simulink model "TestStructure"  (R2022b)
settings: Solver=FixedStepDiscrete  StartTime=0.0  StopTime=300  FixedStep=SampleTime  RelTol=1e-3
InitFcn:
  | SampleTime = 0.001;
  | ButtonValue=0;
  | load("BusConfig.mat");
model workspace (MAT data in the model file):
  Manual_Auto = 1
  Pattern = 1
  Pause_Start = 1
  Stop = 1
  Unlock_Lock = 1
undefined symbols (not defined in the file or in its folder): DiscIntNeverNeededParam
libraries: dspfdesign x4, dspstat3 x4
(part 2 of 3)

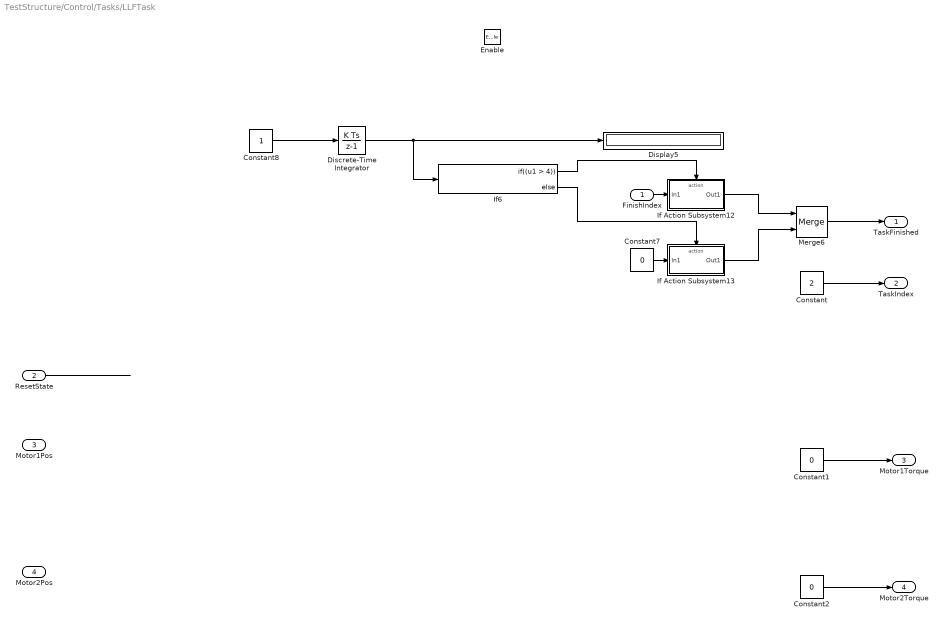
== system TestStructure/Control/Tasks/LLFTask ==
  FinishIndex : Inport
  ResetState : Inport  Port=2
  Motor1Pos : Inport  Port=3
  Motor2Pos : Inport  Port=4
  Enable : EnablePort  StatesWhenEnabling=reset
  Constant : Constant  Value=2
  Constant1 : Constant  Value=0
  Constant2 : Constant  Value=0
  Constant7 : Constant  Value=0  OutDataTypeStr=double
  Constant8 : Constant
  Discrete-Time Integrator : DiscreteIntegrator  SampleTime=-1  ICPrevOutput=DiscIntNeverNeededParam  ICPrevScaledInput=DiscIntNeverNeededParam
  Display5 : Display
  If Action Subsystem12 : Subsystem  TreatAsAtomicUnit=on
  If Action Subsystem13 : Subsystem  TreatAsAtomicUnit=on
  If6 : If  IfExpression=(u1 > 4)
  Merge6 : Merge
  TaskFinished : Outport
  TaskIndex : Outport  Port=2
  Motor1Torque : Outport  Port=3
  Motor2Torque : Outport  Port=4
  wires:
  Merge6/1 -> TaskFinished/1
  If6/1 -> If Action Subsystem12/Action
  Constant8/1 -> Discrete-Time Integrator/1
  If6/2 -> If Action Subsystem13/Action
  Discrete-Time Integrator/1 -> If6/1, Display5/1
  If Action Subsystem13/1(Out1) -> Merge6/2
  FinishIndex/1 -> If Action Subsystem12/1(In1)
  If Action Subsystem12/1(Out1) -> Merge6/1
  Constant7/1 -> If Action Subsystem13/1(In1)
  Constant/1 -> TaskIndex/1
  Constant1/1 -> Motor1Torque/1
  Constant2/1 -> Motor2Torque/1
  ResetState/1 -> ?

== system TestStructure/Control/Tasks/LLWAutoTask ==
  FinishIndex : Inport
  ResetState : Inport  Port=2
  Motor1Pos : Inport  Port=3
  Motor2Pos : Inport  Port=4
  Enable : EnablePort  StatesWhenEnabling=reset
  Constant : Constant  Value=8
  Constant1 : Constant  Value=0
  Constant2 : Constant  Value=0
  Constant7 : Constant  Value=0  OutDataTypeStr=double
  Constant8 : Constant
  Discrete-Time Integrator : DiscreteIntegrator  SampleTime=-1  ICPrevOutput=DiscIntNeverNeededParam  ICPrevScaledInput=DiscIntNeverNeededParam
  Display5 : Display
  If Action Subsystem12 : Subsystem  TreatAsAtomicUnit=on
  If Action Subsystem13 : Subsystem  TreatAsAtomicUnit=on
  If6 : If  IfExpression=(u1 > 4)
  Merge6 : Merge
  TaskFinished : Outport
  TaskIndex : Outport  Port=2
  Motor1Torque : Outport  Port=3
  Motor2Torque : Outport  Port=4
  wires:
  Merge6/1 -> TaskFinished/1
  If6/1 -> If Action Subsystem12/Action
  Constant8/1 -> Discrete-Time Integrator/1
  If6/2 -> If Action Subsystem13/Action
  Discrete-Time Integrator/1 -> If6/1, Display5/1
  If Action Subsystem13/1(Out1) -> Merge6/2
  FinishIndex/1 -> If Action Subsystem12/1(In1)
  If Action Subsystem12/1(Out1) -> Merge6/1
  Constant7/1 -> If Action Subsystem13/1(In1)
  Constant/1 -> TaskIndex/1
  Constant1/1 -> Motor1Torque/1
  Constant2/1 -> Motor2Torque/1
  ResetState/1 -> ?

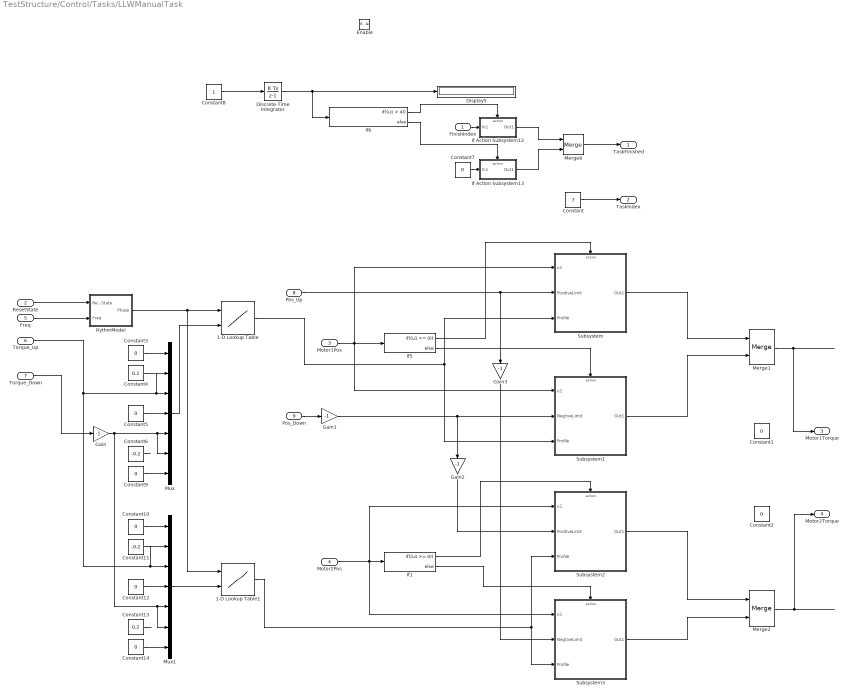
== system TestStructure/Control/Tasks/LLWManualTask ==
  FinishIndex : Inport
  ResetState : Inport  Port=2
  Motor1Pos : Inport  Port=3
  Motor2Pos : Inport  Port=4
  Freq : Inport  Port=5
  Torque_Up : Inport  Port=6
  Torque_Down : Inport  Port=7
  Pos_Up : Inport  Port=8
  Pos_Down : Inport  Port=9
  Enable : EnablePort
  1-D Lookup Table : Lookup_n-D  NumberOfTableDimensions=1  BreakpointsForDimension1=[0;0.2;0.35;0.5;0.65;0.85;1]  TableSource=Input port  Table=[0;0.2;3;0;-3;-0.2;0]  InternalRulePriority=Speed  RndMeth=Simplest
      settings: InputPortMap=u0,p221
  1-D Lookup Table1 : Lookup_n-D  NumberOfTableDimensions=1  BreakpointsForDimension1=[0;0.2;0.35;0.5;0.65;0.85;1]  TableSource=Input port  Table=[0;0.2;3;0;-3;-0.2;0]  InternalRulePriority=Speed  RndMeth=Simplest
      settings: InputPortMap=u0,p221
  Constant : Constant  Value=7
  Constant{1..3,5,9..10,12,14} (8 alike) : Constant  Value=0
  Constant11 : Constant  Value=-0.2
  Constant13 : Constant  Value=0.2
  Constant4 : Constant  Value=0.2
  Constant6 : Constant  Value=-0.2
  Constant7 : Constant  Value=0  OutDataTypeStr=double
  Constant8 : Constant
  Discrete-Time Integrator : DiscreteIntegrator  SampleTime=-1  ICPrevOutput=DiscIntNeverNeededParam  ICPrevScaledInput=DiscIntNeverNeededParam
  Display5 : Display
  Gain{,1..3} (4 alike) : Gain  Gain=-1
  If Action Subsystem12 : Subsystem  TreatAsAtomicUnit=on
  If Action Subsystem13 : Subsystem  TreatAsAtomicUnit=on
  If1 : If  IfExpression=(u1 >= 0)
  If5 : If  IfExpression=(u1 >= 0)
  If6 : If  IfExpression=(u1 > 4)
  Merge1 : Merge
  Merge2 : Merge
  Merge6 : Merge
  Mux : Mux  Inputs=7
  Mux1 : Mux  Inputs=7
  RythmModel : Subsystem
  Subsystem : Subsystem
  Subsystem1 : Subsystem
  Subsystem2 : Subsystem
  Subsystem3 : Subsystem
  TaskFinished : Outport
  TaskIndex : Outport  Port=2
  Motor1Torque : Outport  Port=3
  Motor2Torque : Outport  Port=4
  wires:
  Merge6/1 -> TaskFinished/1
  If6/1 -> If Action Subsystem12/Action
  Constant8/1 -> Discrete-Time Integrator/1
  If6/2 -> If Action Subsystem13/Action
  Discrete-Time Integrator/1 -> If6/1, Display5/1
  If Action Subsystem13/1(Out1) -> Merge6/2
  FinishIndex/1 -> If Action Subsystem12/1(In1)
  If Action Subsystem12/1(Out1) -> Merge6/1
  Constant7/1 -> If Action Subsystem13/1(In1)
  Constant/1 -> TaskIndex/1
  If5/1 -> Subsystem/Action
  Mux1/1 -> 1-D Lookup Table1/2
  Gain3/1 -> Subsystem3/2(NegtiveLimit)
  1-D Lookup Table1/1 -> Subsystem2/3(Profile), Subsystem3/3(Profile)
  Constant12/1 -> Mux1/4
  1-D Lookup Table/1 -> Subsystem1/3(Profile), Subsystem/3(Profile)
  Subsystem/1(Out1) -> Merge1/1
  Mux/1 -> 1-D Lookup Table/2
  Merge1/1 -> Motor1Torque/1
  Merge2/1 -> Motor2Torque/1
  If5/2 -> Subsystem1/Action
  Gain2/1 -> Subsystem2/2(PositiveLimit)
  Gain/1 -> Mux1/5, Mux1/6, Mux/6, Mux/5
  Constant3/1 -> Mux/1
  If1/2 -> Subsystem3/Action
  Subsystem2/1(Out1) -> Merge2/1
  Constant10/1 -> Mux1/1
  Constant5/1 -> Mux/4
  Constant14/1 -> Mux1/7
  ResetState/1 -> RythmModel/1(ResetState)
  Pos_Down/1 -> Gain1/1
  Subsystem1/1(Out1) -> Merge1/2
  If1/1 -> Subsystem2/Action
  RythmModel/1(Phase) -> 1-D Lookup Table1/1, 1-D Lookup Table/1
  Torque_Up/1 -> Mux1/2, Mux1/3, Mux/2, Mux/3
  Subsystem3/1(Out1) -> Merge2/2
  Constant9/1 -> Mux/7
  Constant6/1 -> ?
  Motor1Pos/1 -> Subsystem1/1(u1), If5/1, Subsystem/1(u1)
  Constant13/1 -> ?
  Freq/1 -> RythmModel/2(Freq)
  Torque_Down/1 -> Gain/1
  Constant11/1 -> ?
  Motor2Pos/1 -> Subsystem3/1(u1), Subsystem2/1(u1), If1/1
  Gain1/1 -> Subsystem1/2(NegtiveLimit), Gain2/1
  Constant4/1 -> ?
  Pos_Up/1 -> Subsystem/2(PositiveLimit), Gain3/1

== system TestStructure/Control/Tasks/PauseTask ==
  FinishIndex : Inport
  ResetState : Inport  Port=2
  Motor1Pos : Inport  Port=3
  Motor2Pos : Inport  Port=4
  Enable : EnablePort  StatesWhenEnabling=reset
  Constant : Constant  Value=9
  Constant1 : Constant  Value=0
  Constant2 : Constant  Value=0
  Constant7 : Constant  Value=0  OutDataTypeStr=double
  Constant8 : Constant
  Discrete-Time Integrator : DiscreteIntegrator  SampleTime=-1  ICPrevOutput=DiscIntNeverNeededParam  ICPrevScaledInput=DiscIntNeverNeededParam
  Display5 : Display
  If Action Subsystem12 : Subsystem  TreatAsAtomicUnit=on
  If Action Subsystem13 : Subsystem  TreatAsAtomicUnit=on
  If6 : If  IfExpression=(u1 > 4)
  Merge6 : Merge
  TaskFinished : Outport
  TaskIndex : Outport  Port=2
  Motor1Torque : Outport  Port=3
  Motor2Torque : Outport  Port=4
  wires:
  Merge6/1 -> TaskFinished/1
  If6/1 -> If Action Subsystem12/Action
  Constant8/1 -> Discrete-Time Integrator/1
  If6/2 -> If Action Subsystem13/Action
  Discrete-Time Integrator/1 -> If6/1, Display5/1
  If Action Subsystem13/1(Out1) -> Merge6/2
  FinishIndex/1 -> If Action Subsystem12/1(In1)
  If Action Subsystem12/1(Out1) -> Merge6/1
  Constant7/1 -> If Action Subsystem13/1(In1)
  Constant/1 -> TaskIndex/1
  Constant1/1 -> Motor1Torque/1
  Constant2/1 -> Motor2Torque/1
  ResetState/1 -> ?

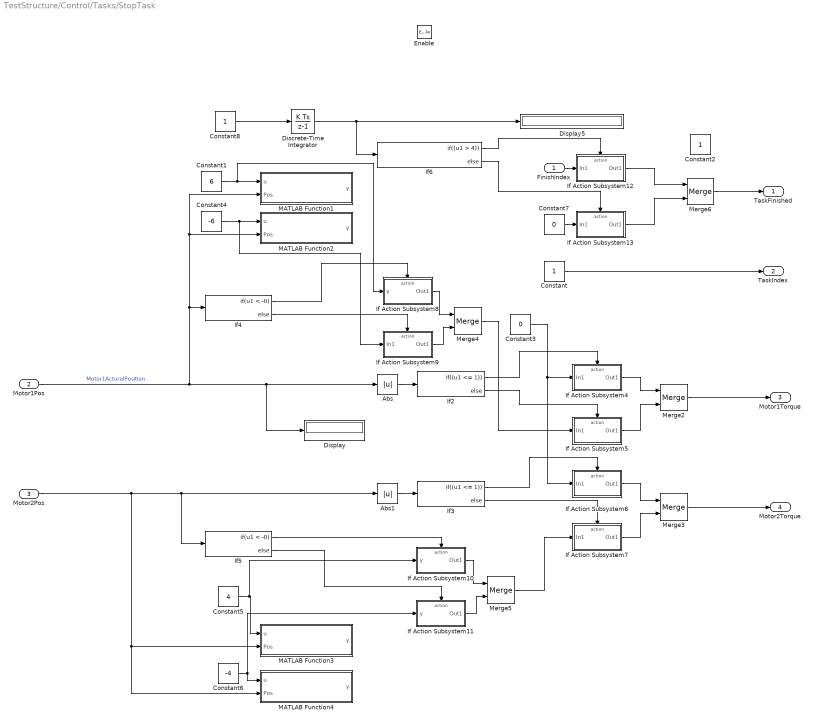
== system TestStructure/Control/Tasks/StopTask ==
  FinishIndex : Inport
  Motor1Pos : Inport  Port=2
  Motor2Pos : Inport  Port=3
  Enable : EnablePort  StatesWhenEnabling=reset
  Abs : Abs  SaturateOnIntegerOverflow=off
  Abs1 : Abs  SaturateOnIntegerOverflow=off
  Constant : Constant
  Constant1 : Constant  Value=6
  Constant2 : Constant
  Constant3 : Constant  Value=0
  Constant4 : Constant  Value=-6
  Constant5 : Constant  Value=4
  Constant6 : Constant  Value=-4
  Constant7 : Constant  Value=0  OutDataTypeStr=double
  Constant8 : Constant
  Discrete-Time Integrator : DiscreteIntegrator  SampleTime=-1  ICPrevOutput=DiscIntNeverNeededParam  ICPrevScaledInput=DiscIntNeverNeededParam
  Display : Display
  Display5 : Display
  If Action Subsystem10 : Subsystem  TreatAsAtomicUnit=on
  If Action Subsystem11 : Subsystem  TreatAsAtomicUnit=on
  If Action Subsystem12 : Subsystem  TreatAsAtomicUnit=on
  If Action Subsystem13 : Subsystem  TreatAsAtomicUnit=on
  If Action Subsystem4 : Subsystem  TreatAsAtomicUnit=on
  If Action Subsystem5 : Subsystem  TreatAsAtomicUnit=on
  If Action Subsystem6 : Subsystem  TreatAsAtomicUnit=on
  If Action Subsystem7 : Subsystem  TreatAsAtomicUnit=on
  If Action Subsystem8 : Subsystem  TreatAsAtomicUnit=on
  If Action Subsystem9 : Subsystem  TreatAsAtomicUnit=on
  If2 : If  IfExpression=(u1 <= 1)
  If3 : If  IfExpression=(u1 <= 1)
  If4 : If  IfExpression=u1 < -0
  If5 : If  IfExpression=u1 < -0
  If6 : If  IfExpression=(u1 > 4)
  MATLAB Function1 : MATLAB Function  TreatAsAtomicUnit=on
  MATLAB Function2 : MATLAB Function  TreatAsAtomicUnit=on
  MATLAB Function3 : MATLAB Function  TreatAsAtomicUnit=on
  MATLAB Function4 : MATLAB Function  TreatAsAtomicUnit=on
  Merge{2..6} (5 alike) : Merge
  TaskFinished : Outport
  TaskIndex : Outport  Port=2
  Motor1Torque : Outport  Port=3
  Motor2Torque : Outport  Port=4
  wires:
  Merge6/1 -> TaskFinished/1
  If6/1 -> If Action Subsystem12/Action
  If2/1 -> If Action Subsystem4/Action
  Constant1/1 -> If Action Subsystem8/1(y), MATLAB Function1/1(u)
  If Action Subsystem11/1(Out1) -> Merge5/2
  Constant5/1 -> If Action Subsystem10/1(y), MATLAB Function3/1(u)
  If5/2 -> If Action Subsystem11/Action
  If4/2 -> If Action Subsystem9/Action
  If Action Subsystem8/1(Out1) -> Merge4/1
  If3/2 -> If Action Subsystem7/Action
  If4/1 -> If Action Subsystem8/Action
  If Action Subsystem10/1(Out1) -> Merge5/1
  Constant8/1 -> Discrete-Time Integrator/1
  If2/2 -> If Action Subsystem5/Action
  Merge5/1 -> If Action Subsystem7/1(In1)
  Merge3/1 -> Motor2Torque/1
  If5/1 -> If Action Subsystem10/Action
  Abs/1 -> If2/1
  Merge4/1 -> If Action Subsystem5/1(In1)
  Merge2/1 -> Motor1Torque/1
  Constant3/1 -> If Action Subsystem6/1(In1), If Action Subsystem4/1(In1)
  If Action Subsystem9/1(Out1) -> Merge4/2
  Motor2Pos/1 -> MATLAB Function4/2(Pos), MATLAB Function3/2(Pos), If5/1, Abs1/1
  Motor1Pos/1 -> MATLAB Function2/2(Pos), MATLAB Function1/2(Pos), If4/1, Abs/1, Display/1  "Motor1ActuralPosition"
  If6/2 -> If Action Subsystem13/Action
  Abs1/1 -> If3/1
  Discrete-Time Integrator/1 -> If6/1, Display5/1
  If Action Subsystem13/1(Out1) -> Merge6/2
  If Action Subsystem7/1(Out1) -> Merge3/2
  FinishIndex/1 -> If Action Subsystem12/1(In1)
  If Action Subsystem12/1(Out1) -> Merge6/1
  If Action Subsystem6/1(Out1) -> Merge3/1
  If Action Subsystem4/1(Out1) -> Merge2/1
  If3/1 -> If Action Subsystem6/Action
  If Action Subsystem5/1(Out1) -> Merge2/2
  Constant7/1 -> If Action Subsystem13/1(In1)
  Constant4/1 -> If Action Subsystem9/1(In1), MATLAB Function2/1(u)
  Constant6/1 -> If Action Subsystem11/1(y), MATLAB Function4/1(u)
  Constant/1 -> TaskIndex/1

== system TestStructure/Control/Tasks/ULLockTask ==
  FinishIndex : Inport
  ResetState : Inport  Port=2
  Motor3Pos : Inport  Port=3
  Motor4Pos : Inport  Port=4
  Enable : EnablePort  StatesWhenEnabling=reset
  Constant : Constant  Value=2
  Constant1 : Constant  Value=0
  Constant2 : Constant  Value=0
  Constant7 : Constant  Value=0  OutDataTypeStr=double
  Constant8 : Constant
  Discrete-Time Integrator : DiscreteIntegrator  SampleTime=-1  ICPrevOutput=DiscIntNeverNeededParam  ICPrevScaledInput=DiscIntNeverNeededParam
  Display5 : Display
  If Action Subsystem12 : Subsystem  TreatAsAtomicUnit=on
  If Action Subsystem13 : Subsystem  TreatAsAtomicUnit=on
  If6 : If  IfExpression=(u1 > 4)
  Merge6 : Merge
  TaskFinished : Outport
  TaskIndex : Outport  Port=2
  Motor3Torque : Outport  Port=3
  Motor4Torque : Outport  Port=4
  wires:
  Merge6/1 -> TaskFinished/1
  If6/1 -> If Action Subsystem12/Action
  Constant8/1 -> Discrete-Time Integrator/1
  If6/2 -> If Action Subsystem13/Action
  Discrete-Time Integrator/1 -> If6/1, Display5/1
  If Action Subsystem13/1(Out1) -> Merge6/2
  FinishIndex/1 -> If Action Subsystem12/1(In1)
  If Action Subsystem12/1(Out1) -> Merge6/1
  Constant7/1 -> If Action Subsystem13/1(In1)
  Constant/1 -> TaskIndex/1
  Constant1/1 -> Motor3Torque/1
  Constant2/1 -> Motor4Torque/1
  ResetState/1 -> ?

== system TestStructure/Control/Tasks/ULUnLockTask ==
  FinishIndex : Inport
  ResetState : Inport  Port=2
  Motor3Pos : Inport  Port=3
  Motor4Pos : Inport  Port=4
  Enable : EnablePort  StatesWhenEnabling=reset
  Constant : Constant
  Constant1 : Constant  Value=0
  Constant2 : Constant  Value=0
  Constant7 : Constant  Value=0  OutDataTypeStr=double
  Constant8 : Constant
  Discrete-Time Integrator : DiscreteIntegrator  SampleTime=-1  ICPrevOutput=DiscIntNeverNeededParam  ICPrevScaledInput=DiscIntNeverNeededParam
  Display5 : Display
  If Action Subsystem12 : Subsystem  TreatAsAtomicUnit=on
  If Action Subsystem13 : Subsystem  TreatAsAtomicUnit=on
  If6 : If  IfExpression=(u1 > 4)
  Merge6 : Merge
  TaskFinished : Outport
  TaskIndex : Outport  Port=2
  Motor3Torque : Outport  Port=3
  Motor4Torque : Outport  Port=4
  wires:
  Merge6/1 -> TaskFinished/1
  If6/1 -> If Action Subsystem12/Action
  Constant8/1 -> Discrete-Time Integrator/1
  If6/2 -> If Action Subsystem13/Action
  Discrete-Time Integrator/1 -> If6/1, Display5/1
  If Action Subsystem13/1(Out1) -> Merge6/2
  FinishIndex/1 -> If Action Subsystem12/1(In1)
  If Action Subsystem12/1(Out1) -> Merge6/1
  Constant7/1 -> If Action Subsystem13/1(In1)
  Constant/1 -> TaskIndex/1
  Constant1/1 -> Motor3Torque/1
  Constant2/1 -> Motor4Torque/1
  ResetState/1 -> ?

== system TestStructure/Control/PanelController/Display_State_1_Enable/Subsystem ==
  Case : Inport
  Case Default : Inport  Port=2
  Constant : Constant
  Constant1 : Constant  Value=0
  Constant2 : Constant  Value=TaskIndex
  Merge : Merge
  Switch Case Action Subsystem : Subsystem  TreatAsAtomicUnit=on
  Switch Case Action Subsystem1 : Subsystem  TreatAsAtomicUnit=on
  Enable : Outport
  FinishIndex : Outport  Port=2
  wires:
  Constant/1 -> Switch Case Action Subsystem/1(In1)
  Case/1 -> Switch Case Action Subsystem/Action
  Switch Case Action Subsystem/1(Out1) -> Merge/1
  Merge/1 -> Enable/1
  Case Default/1 -> Switch Case Action Subsystem1/Action
  Constant1/1 -> Switch Case Action Subsystem1/1(In1)
  Switch Case Action Subsystem1/1(Default) -> Merge/2
  Constant2/1 -> FinishIndex/1

== system TestStructure/Control/PanelController/Display_State_2_Enable/Subsystem ==
  Case : Inport
  Case Default : Inport  Port=2
  Constant : Constant
  Constant1 : Constant  Value=0
  Constant2 : Constant  Value=TaskIndex
  Merge : Merge
  Switch Case Action Subsystem : Subsystem  TreatAsAtomicUnit=on
  Switch Case Action Subsystem1 : Subsystem  TreatAsAtomicUnit=on
  Enable : Outport
  FinishIndex : Outport  Port=2
  wires:
  Constant/1 -> Switch Case Action Subsystem/1(In1)
  Case/1 -> Switch Case Action Subsystem/Action
  Switch Case Action Subsystem/1(Out1) -> Merge/1
  Merge/1 -> Enable/1
  Case Default/1 -> Switch Case Action Subsystem1/Action
  Constant1/1 -> Switch Case Action Subsystem1/1(In1)
  Switch Case Action Subsystem1/1(Default) -> Merge/2
  Constant2/1 -> FinishIndex/1

== system TestStructure/Control/PanelController/Display_State_3_Enable/Subsystem ==
  Case : Inport
  Case Default : Inport  Port=2
  Constant : Constant
  Constant1 : Constant  Value=0
  Constant2 : Constant  Value=TaskIndex
  Merge : Merge
  Switch Case Action Subsystem : Subsystem  TreatAsAtomicUnit=on
  Switch Case Action Subsystem1 : Subsystem  TreatAsAtomicUnit=on
  Enable : Outport
  FinishIndex : Outport  Port=2
  wires:
  Constant/1 -> Switch Case Action Subsystem/1(In1)
  Case/1 -> Switch Case Action Subsystem/Action
  Switch Case Action Subsystem/1(Out1) -> Merge/1
  Merge/1 -> Enable/1
  Case Default/1 -> Switch Case Action Subsystem1/Action
  Constant1/1 -> Switch Case Action Subsystem1/1(In1)
  Switch Case Action Subsystem1/1(Default) -> Merge/2
  Constant2/1 -> FinishIndex/1

== system TestStructure/Control/PanelController/Display_State_4_Enable/Subsystem ==
  Case : Inport
  Case Default : Inport  Port=2
  Constant : Constant
  Constant1 : Constant  Value=0
  Constant2 : Constant  Value=TaskIndex
  Merge : Merge
  Switch Case Action Subsystem : Subsystem  TreatAsAtomicUnit=on
  Switch Case Action Subsystem1 : Subsystem  TreatAsAtomicUnit=on
  Enable : Outport
  FinishIndex : Outport  Port=2
  wires:
  Constant/1 -> Switch Case Action Subsystem/1(In1)
  Case/1 -> Switch Case Action Subsystem/Action
  Switch Case Action Subsystem/1(Out1) -> Merge/1
  Merge/1 -> Enable/1
  Case Default/1 -> Switch Case Action Subsystem1/Action
  Constant1/1 -> Switch Case Action Subsystem1/1(In1)
  Switch Case Action Subsystem1/1(Default) -> Merge/2
  Constant2/1 -> FinishIndex/1

== system TestStructure/Control/PanelController/LLTaskControl_State_1_Enable/Subsystem ==
  Case : Inport
  Case Default : Inport  Port=2
  Constant : Constant
  Constant1 : Constant  Value=0
  Constant2 : Constant  Value=TaskIndex
  Merge : Merge
  Switch Case Action Subsystem : Subsystem  TreatAsAtomicUnit=on
  Switch Case Action Subsystem1 : Subsystem  TreatAsAtomicUnit=on
  Enable : Outport
  FinishIndex : Outport  Port=2
  wires:
  Constant/1 -> Switch Case Action Subsystem/1(In1)
  Case/1 -> Switch Case Action Subsystem/Action
  Switch Case Action Subsystem/1(Out1) -> Merge/1
  Merge/1 -> Enable/1
  Case Default/1 -> Switch Case Action Subsystem1/Action
  Constant1/1 -> Switch Case Action Subsystem1/1(In1)
  Switch Case Action Subsystem1/1(Default) -> Merge/2
  Constant2/1 -> FinishIndex/1

== system TestStructure/Control/PanelController/LLTaskControl_State_2_Enable/Subsystem ==
  Case : Inport
  Case Default : Inport  Port=2
  Constant : Constant
  Constant1 : Constant  Value=0
  Constant2 : Constant  Value=TaskIndex
  Merge : Merge
  Switch Case Action Subsystem : Subsystem  TreatAsAtomicUnit=on
  Switch Case Action Subsystem1 : Subsystem  TreatAsAtomicUnit=on
  Enable : Outport
  FinishIndex : Outport  Port=2
  wires:
  Constant/1 -> Switch Case Action Subsystem/1(In1)
  Case/1 -> Switch Case Action Subsystem/Action
  Switch Case Action Subsystem/1(Out1) -> Merge/1
  Merge/1 -> Enable/1
  Case Default/1 -> Switch Case Action Subsystem1/Action
  Constant1/1 -> Switch Case Action Subsystem1/1(In1)
  Switch Case Action Subsystem1/1(Default) -> Merge/2
  Constant2/1 -> FinishIndex/1

== system TestStructure/Control/PanelController/LLTaskControl_State_3_Enable/Subsystem ==
  Case : Inport
  Case Default : Inport  Port=2
  Constant : Constant
  Constant1 : Constant  Value=0
  Constant2 : Constant  Value=TaskIndex
  Merge : Merge
  Switch Case Action Subsystem : Subsystem  TreatAsAtomicUnit=on
  Switch Case Action Subsystem1 : Subsystem  TreatAsAtomicUnit=on
  Enable : Outport
  FinishIndex : Outport  Port=2
  wires:
  Constant/1 -> Switch Case Action Subsystem/1(In1)
  Case/1 -> Switch Case Action Subsystem/Action
  Switch Case Action Subsystem/1(Out1) -> Merge/1
  Merge/1 -> Enable/1
  Case Default/1 -> Switch Case Action Subsystem1/Action
  Constant1/1 -> Switch Case Action Subsystem1/1(In1)
  Switch Case Action Subsystem1/1(Default) -> Merge/2
  Constant2/1 -> FinishIndex/1

== system TestStructure/Control/PanelController/LLTaskControl_State_4_Enable/Subsystem ==
  Case : Inport
  Case Default : Inport  Port=2
  Constant : Constant
  Constant1 : Constant  Value=0
  Constant2 : Constant  Value=TaskIndex
  Merge : Merge
  Switch Case Action Subsystem : Subsystem  TreatAsAtomicUnit=on
  Switch Case Action Subsystem1 : Subsystem  TreatAsAtomicUnit=on
  Enable : Outport
  FinishIndex : Outport  Port=2
  wires:
  Constant/1 -> Switch Case Action Subsystem/1(In1)
  Case/1 -> Switch Case Action Subsystem/Action
  Switch Case Action Subsystem/1(Out1) -> Merge/1
  Merge/1 -> Enable/1
  Case Default/1 -> Switch Case Action Subsystem1/Action
  Constant1/1 -> Switch Case Action Subsystem1/1(In1)
  Switch Case Action Subsystem1/1(Default) -> Merge/2
  Constant2/1 -> FinishIndex/1

== system TestStructure/Control/PanelController/LLTaskControl_State_5_Enable/Subsystem ==
  Case : Inport
  Case Default : Inport  Port=2
  Constant : Constant
  Constant1 : Constant  Value=0
  Constant2 : Constant  Value=TaskIndex
  Merge : Merge
  Switch Case Action Subsystem : Subsystem  TreatAsAtomicUnit=on
  Switch Case Action Subsystem1 : Subsystem  TreatAsAtomicUnit=on
  Enable : Outport
  FinishIndex : Outport  Port=2
  wires:
  Constant/1 -> Switch Case Action Subsystem/1(In1)
  Case/1 -> Switch Case Action Subsystem/Action
  Switch Case Action Subsystem/1(Out1) -> Merge/1
  Merge/1 -> Enable/1
  Case Default/1 -> Switch Case Action Subsystem1/Action
  Constant1/1 -> Switch Case Action Subsystem1/1(In1)
  Switch Case Action Subsystem1/1(Default) -> Merge/2
  Constant2/1 -> FinishIndex/1

== system TestStructure/Control/PanelController/LLTaskControl_State_6_Enable/Subsystem ==
  Case : Inport
  Case Default : Inport  Port=2
  Constant : Constant
  Constant1 : Constant  Value=0
  Constant2 : Constant  Value=TaskIndex
  Merge : Merge
  Switch Case Action Subsystem : Subsystem  TreatAsAtomicUnit=on
  Switch Case Action Subsystem1 : Subsystem  TreatAsAtomicUnit=on
  Enable : Outport
  FinishIndex : Outport  Port=2
  wires:
  Constant/1 -> Switch Case Action Subsystem/1(In1)
  Case/1 -> Switch Case Action Subsystem/Action
  Switch Case Action Subsystem/1(Out1) -> Merge/1
  Merge/1 -> Enable/1
  Case Default/1 -> Switch Case Action Subsystem1/Action
  Constant1/1 -> Switch Case Action Subsystem1/1(In1)
  Switch Case Action Subsystem1/1(Default) -> Merge/2
  Constant2/1 -> FinishIndex/1

== system TestStructure/Control/PanelController/LLTaskControl_State_7_Enable/Subsystem ==
  Case : Inport
  Case Default : Inport  Port=2
  Constant : Constant
  Constant1 : Constant  Value=0
  Constant2 : Constant  Value=TaskIndex
  Merge : Merge
  Switch Case Action Subsystem : Subsystem  TreatAsAtomicUnit=on
  Switch Case Action Subsystem1 : Subsystem  TreatAsAtomicUnit=on
  Enable : Outport
  FinishIndex : Outport  Port=2
  wires:
  Constant/1 -> Switch Case Action Subsystem/1(In1)
  Case/1 -> Switch Case Action Subsystem/Action
  Switch Case Action Subsystem/1(Out1) -> Merge/1
  Merge/1 -> Enable/1
  Case Default/1 -> Switch Case Action Subsystem1/Action
  Constant1/1 -> Switch Case Action Subsystem1/1(In1)
  Switch Case Action Subsystem1/1(Default) -> Merge/2
  Constant2/1 -> FinishIndex/1

== system TestStructure/Control/PanelController/LLTaskControl_State_8_Enable/Subsystem ==
  Case : Inport
  Case Default : Inport  Port=2
  Constant : Constant
  Constant1 : Constant  Value=0
  Constant2 : Constant  Value=TaskIndex
  Merge : Merge
  Switch Case Action Subsystem : Subsystem  TreatAsAtomicUnit=on
  Switch Case Action Subsystem1 : Subsystem  TreatAsAtomicUnit=on
  Enable : Outport
  FinishIndex : Outport  Port=2
  wires:
  Constant/1 -> Switch Case Action Subsystem/1(In1)
  Case/1 -> Switch Case Action Subsystem/Action
  Switch Case Action Subsystem/1(Out1) -> Merge/1
  Merge/1 -> Enable/1
  Case Default/1 -> Switch Case Action Subsystem1/Action
  Constant1/1 -> Switch Case Action Subsystem1/1(In1)
  Switch Case Action Subsystem1/1(Default) -> Merge/2
  Constant2/1 -> FinishIndex/1

== system TestStructure/Control/PanelController/LLTaskControl_State_9_Enable/Subsystem ==
  Case : Inport
  Case Default : Inport  Port=2
  Constant : Constant
  Constant1 : Constant  Value=0
  Constant2 : Constant  Value=TaskIndex
  Merge : Merge
  Switch Case Action Subsystem : Subsystem  TreatAsAtomicUnit=on
  Switch Case Action Subsystem1 : Subsystem  TreatAsAtomicUnit=on
  Enable : Outport
  FinishIndex : Outport  Port=2
  wires:
  Constant/1 -> Switch Case Action Subsystem/1(In1)
  Case/1 -> Switch Case Action Subsystem/Action
  Switch Case Action Subsystem/1(Out1) -> Merge/1
  Merge/1 -> Enable/1
  Case Default/1 -> Switch Case Action Subsystem1/Action
  Constant1/1 -> Switch Case Action Subsystem1/1(In1)
  Switch Case Action Subsystem1/1(Default) -> Merge/2
  Constant2/1 -> FinishIndex/1

== system TestStructure/Control/PanelController/ULTaskControl_State_1_Enable/Subsystem ==
  Case : Inport
  Case Default : Inport  Port=2
  Constant : Constant
  Constant1 : Constant  Value=0
  Constant2 : Constant  Value=TaskIndex
  Merge : Merge
  Switch Case Action Subsystem : Subsystem  TreatAsAtomicUnit=on
  Switch Case Action Subsystem1 : Subsystem  TreatAsAtomicUnit=on
  Enable : Outport
  FinishIndex : Outport  Port=2
  wires:
  Constant/1 -> Switch Case Action Subsystem/1(In1)
  Case/1 -> Switch Case Action Subsystem/Action
  Switch Case Action Subsystem/1(Out1) -> Merge/1
  Merge/1 -> Enable/1
  Case Default/1 -> Switch Case Action Subsystem1/Action
  Constant1/1 -> Switch Case Action Subsystem1/1(In1)
  Switch Case Action Subsystem1/1(Default) -> Merge/2
  Constant2/1 -> FinishIndex/1

== system TestStructure/Control/PanelController/ULTaskControl_State_2_Enable/Subsystem ==
  Case : Inport
  Case Default : Inport  Port=2
  Constant : Constant
  Constant1 : Constant  Value=0
  Constant2 : Constant  Value=TaskIndex
  Merge : Merge
  Switch Case Action Subsystem : Subsystem  TreatAsAtomicUnit=on
  Switch Case Action Subsystem1 : Subsystem  TreatAsAtomicUnit=on
  Enable : Outport
  FinishIndex : Outport  Port=2
  wires:
  Constant/1 -> Switch Case Action Subsystem/1(In1)
  Case/1 -> Switch Case Action Subsystem/Action
  Switch Case Action Subsystem/1(Out1) -> Merge/1
  Merge/1 -> Enable/1
  Case Default/1 -> Switch Case Action Subsystem1/Action
  Constant1/1 -> Switch Case Action Subsystem1/1(In1)
  Switch Case Action Subsystem1/1(Default) -> Merge/2
  Constant2/1 -> FinishIndex/1

== system TestStructure/Control/Tasks/LLBAutoTask/If Action Subsystem12 ==
  In1 : Inport
  Action Port : ActionPort  ActionPortLabel=if((u1 > 4))
  Out1 : Outport
  wires:
  In1/1 -> Out1/1

== system TestStructure/Control/Tasks/LLBAutoTask/If Action Subsystem13 ==
  In1 : Inport
  Action Port : ActionPort  ActionPortLabel=else
  Out1 : Outport
  wires:
  In1/1 -> Out1/1

== system TestStructure/Control/Tasks/LLBManualTask/If Action Subsystem12 ==
  In1 : Inport
  Action Port : ActionPort  ActionPortLabel=if((u1 > 4))
  Out1 : Outport
  wires:
  In1/1 -> Out1/1

== system TestStructure/Control/Tasks/LLBManualTask/If Action Subsystem13 ==
  In1 : Inport
  Action Port : ActionPort  ActionPortLabel=else
  Out1 : Outport
  wires:
  In1/1 -> Out1/1

== system TestStructure/Control/Tasks/LLBManualTask/RythmModel ==
  ResetState : Inport
  Freq : Inport  Port=2
  Chart : Stateflow chart  TreatAsAtomicUnit=on
      settings: PortSchema="{\"entries\":[{\"content\":{\"sides\":[{\"content\":{\"connectorIds\":[\"In2\",\"In3\"]},\"type\":\"ConnectorPlacement.EquallySpacedRectSide\",\"uuid\":\"12385952-88cf-46bd-a9c8-6e14cd4b2c44\"},{\"content\":{\"connectorIds\":[\"Out1\",\"Out2\"],\"side\":\"RIGHT\"},\"type\":\"ConnectorPlacement.EquallySpacedRectSide\",\"uuid\":\"6211c7ba-d55b-4eba-bf5b-7c1649feb09f\"},{\"content\":{\"connectorIds\":[\"In1\"],\"side\":\"TOP\"},\"type\":\"ConnectorPlacement.EquallySpacedRectSide\",\"uuid\":\"17e15bab-f9dc-4c89-b15c-8ab250c59318\"},{\"content\":{\"connectorIds\":[\"In4\"],\"side\":\"BOTTOM\"},\"type\":\"ConnectorPlacement.EquallySpacedRectSide\",\"uuid\":\"029db472-06b3-40cc-b087-bfb8d6677823\"}]},\"type\":\"ConnectorPlacement.EquallySpacedConnector\",\"uuid\":\"9e8824a0-257a-42b2-87f9-63b657fce5f4\"}],\"packageUris\":[\"http://schema.mathworks.com/mf0/Connector/R2020b\"],\"version\":\"1.0\"}"
  Constant3 : Constant  Value=SampleTime
  Discrete-Time Integrator1 : DiscreteIntegrator  ExternalReset=rising  SampleTime=-1  LimitOutput=on  UpperSaturationLimit=1  LowerSaturationLimit=0  ICPrevOutput=DiscIntNeverNeededParam  ICPrevScaledInput=DiscIntNeverNeededParam
  Math Function : Math  Operator=reciprocal
  Memory : Memory
  Phase : Outport
  wires:
  Constant3/1 -> Chart/3(SampleTime)
  Discrete-Time Integrator1/1 -> Phase/1, Memory/1
  Chart/1(Input) -> Discrete-Time Integrator1/1
  Chart/2(Reset) -> Discrete-Time Integrator1/2
  Math Function/1 -> Chart/2(Period)
  Freq/1 -> Math Function/1
  Memory/1 -> Chart/4(IntVal)
  ResetState/1 -> Chart/1(ResetState)

== system TestStructure/Control/Tasks/LLBManualTask/Subsystem ==
  u1 : Inport
  PositiveLimit : Inport  Port=2
  Profile : Inport  Port=3
  Action Port : ActionPort  ActionPortLabel=if((u1 >= 0))
  Constant15 : Constant  Value=0
  If Action Subsystem4 : Subsystem  TreatAsAtomicUnit=on
  If Action Subsystem5 : Subsystem  TreatAsAtomicUnit=on
  If2 : If  NumInputs=2  IfExpression=(u1 <= u2)
  Merge1 : Merge
  MinMax : MinMax  Inputs=2
  Out1 : Outport
  wires:
  MinMax/1 -> If Action Subsystem4/1(In1)
  Profile/1 -> MinMax/2, If Action Subsystem5/1(In1)
  If2/1 -> If Action Subsystem5/Action
  u1/1 -> If2/1
  If2/2 -> If Action Subsystem4/Action
  If Action Subsystem5/1(Out1) -> Merge1/2
  If Action Subsystem4/1(Out1) -> Merge1/1
  PositiveLimit/1 -> If2/2
  Merge1/1 -> Out1/1
  Constant15/1 -> MinMax/1

== system TestStructure/Control/Tasks/LLBManualTask/Subsystem1 ==
  u1 : Inport
  NegtiveLimit : Inport  Port=2
  Profile : Inport  Port=3
  Action Port : ActionPort  ActionPortLabel=else
  Constant16 : Constant  Value=0
  If Action Subsystem1 : Subsystem  TreatAsAtomicUnit=on
  If Action Subsystem2 : Subsystem  TreatAsAtomicUnit=on
  If1 : If  NumInputs=2  IfExpression=(u1 >= u2)
  Merge1 : Merge
  MinMax : MinMax  Function=max  Inputs=2
  Out1 : Outport
  wires:
  Profile/1 -> MinMax/2, If Action Subsystem2/1(Motor1Pos)
  u1/1 -> If1/1
  If Action Subsystem2/1(Out1) -> Merge1/2
  If Action Subsystem1/1(Out1) -> Merge1/1
  NegtiveLimit/1 -> If1/2
  Merge1/1 -> Out1/1
  If1/2 -> If Action Subsystem1/Action
  If1/1 -> If Action Subsystem2/Action
  MinMax/1 -> If Action Subsystem1/1(In1)
  Constant16/1 -> MinMax/1

== system TestStructure/Control/Tasks/LLBManualTask/Subsystem2 ==
  u1 : Inport
  PositiveLimit : Inport  Port=2
  Profile : Inport  Port=3
  Action Port : ActionPort  ActionPortLabel=if((u1 >= 0))
  Constant15 : Constant  Value=0
  If Action Subsystem4 : Subsystem  TreatAsAtomicUnit=on
  If Action Subsystem5 : Subsystem  TreatAsAtomicUnit=on
  If2 : If  NumInputs=2  IfExpression=(u1 <= u2)
  Merge1 : Merge
  MinMax : MinMax  Inputs=2
  Out1 : Outport
  wires:
  MinMax/1 -> If Action Subsystem4/1(In1)
  Profile/1 -> MinMax/2, If Action Subsystem5/1(In1)
  If2/1 -> If Action Subsystem5/Action
  u1/1 -> If2/1
  If2/2 -> If Action Subsystem4/Action
  If Action Subsystem5/1(Out1) -> Merge1/2
  If Action Subsystem4/1(Out1) -> Merge1/1
  PositiveLimit/1 -> If2/2
  Merge1/1 -> Out1/1
  Constant15/1 -> MinMax/1

== system TestStructure/Control/Tasks/LLBManualTask/Subsystem3 ==
  u1 : Inport
  NegtiveLimit : Inport  Port=2
  Profile : Inport  Port=3
  Action Port : ActionPort  ActionPortLabel=else
  Constant16 : Constant  Value=0
  If Action Subsystem1 : Subsystem  TreatAsAtomicUnit=on
  If Action Subsystem2 : Subsystem  TreatAsAtomicUnit=on
  If1 : If  NumInputs=2  IfExpression=(u1 >= u2)
  Merge1 : Merge
  MinMax : MinMax  Function=max  Inputs=2
  Out1 : Outport
  wires:
  Profile/1 -> MinMax/2, If Action Subsystem2/1(Motor1Pos)
  u1/1 -> If1/1
  If Action Subsystem2/1(Out1) -> Merge1/2
  If Action Subsystem1/1(Out1) -> Merge1/1
  NegtiveLimit/1 -> If1/2
  Merge1/1 -> Out1/1
  If1/2 -> If Action Subsystem1/Action
  If1/1 -> If Action Subsystem2/Action
  MinMax/1 -> If Action Subsystem1/1(In1)
  Constant16/1 -> MinMax/1

== system TestStructure/Control/Tasks/LLFKAutoTask/If Action Subsystem12 ==
  In1 : Inport
  Action Port : ActionPort  ActionPortLabel=if((u1 > 4))
  Out1 : Outport
  wires:
  In1/1 -> Out1/1

== system TestStructure/Control/Tasks/LLFKAutoTask/If Action Subsystem13 ==
  In1 : Inport
  Action Port : ActionPort  ActionPortLabel=else
  Out1 : Outport
  wires:
  In1/1 -> Out1/1

== system TestStructure/Control/Tasks/LLFKManualTask/If Action Subsystem12 ==
  In1 : Inport
  Action Port : ActionPort  ActionPortLabel=if((u1 > 4))
  Out1 : Outport
  wires:
  In1/1 -> Out1/1

== system TestStructure/Control/Tasks/LLFKManualTask/If Action Subsystem13 ==
  In1 : Inport
  Action Port : ActionPort  ActionPortLabel=else
  Out1 : Outport
  wires:
  In1/1 -> Out1/1

== system TestStructure/Control/Tasks/LLFTask/If Action Subsystem12 ==
  In1 : Inport
  Action Port : ActionPort  ActionPortLabel=if((u1 > 4))
  Out1 : Outport
  wires:
  In1/1 -> Out1/1

== system TestStructure/Control/Tasks/LLFTask/If Action Subsystem13 ==
  In1 : Inport
  Action Port : ActionPort  ActionPortLabel=else
  Out1 : Outport
  wires:
  In1/1 -> Out1/1

== system TestStructure/Control/Tasks/LLWAutoTask/If Action Subsystem12 ==
  In1 : Inport
  Action Port : ActionPort  ActionPortLabel=if((u1 > 4))
  Out1 : Outport
  wires:
  In1/1 -> Out1/1

== system TestStructure/Control/Tasks/LLWAutoTask/If Action Subsystem13 ==
  In1 : Inport
  Action Port : ActionPort  ActionPortLabel=else
  Out1 : Outport
  wires:
  In1/1 -> Out1/1

== system TestStructure/Control/Tasks/LLWManualTask/If Action Subsystem12 ==
  In1 : Inport
  Action Port : ActionPort  ActionPortLabel=if((u1 > 4))
  Out1 : Outport
  wires:
  In1/1 -> Out1/1

== system TestStructure/Control/Tasks/LLWManualTask/If Action Subsystem13 ==
  In1 : Inport
  Action Port : ActionPort  ActionPortLabel=else
  Out1 : Outport
  wires:
  In1/1 -> Out1/1

== system TestStructure/Control/Tasks/LLWManualTask/RythmModel ==
  ResetState : Inport
  Freq : Inport  Port=2
  Chart : Stateflow chart  TreatAsAtomicUnit=on
      settings: PortSchema="{\"entries\":[{\"content\":{\"sides\":[{\"content\":{\"connectorIds\":[\"In2\",\"In3\"]},\"type\":\"ConnectorPlacement.EquallySpacedRectSide\",\"uuid\":\"12385952-88cf-46bd-a9c8-6e14cd4b2c44\"},{\"content\":{\"connectorIds\":[\"Out1\",\"Out2\"],\"side\":\"RIGHT\"},\"type\":\"ConnectorPlacement.EquallySpacedRectSide\",\"uuid\":\"6211c7ba-d55b-4eba-bf5b-7c1649feb09f\"},{\"content\":{\"connectorIds\":[\"In1\"],\"side\":\"TOP\"},\"type\":\"ConnectorPlacement.EquallySpacedRectSide\",\"uuid\":\"17e15bab-f9dc-4c89-b15c-8ab250c59318\"},{\"content\":{\"connectorIds\":[\"In4\"],\"side\":\"BOTTOM\"},\"type\":\"ConnectorPlacement.EquallySpacedRectSide\",\"uuid\":\"029db472-06b3-40cc-b087-bfb8d6677823\"}]},\"type\":\"ConnectorPlacement.EquallySpacedConnector\",\"uuid\":\"9e8824a0-257a-42b2-87f9-63b657fce5f4\"}],\"packageUris\":[\"http://schema.mathworks.com/mf0/Connector/R2020b\"],\"version\":\"1.0\"}"
  Constant3 : Constant  Value=SampleTime
  Discrete-Time Integrator1 : DiscreteIntegrator  ExternalReset=rising  SampleTime=-1  LimitOutput=on  UpperSaturationLimit=1  LowerSaturationLimit=0  ICPrevOutput=DiscIntNeverNeededParam  ICPrevScaledInput=DiscIntNeverNeededParam
  Math Function : Math  Operator=reciprocal
  Memory : Memory
  Phase : Outport
  wires:
  Constant3/1 -> Chart/3(SampleTime)
  Discrete-Time Integrator1/1 -> Phase/1, Memory/1
  Chart/1(Input) -> Discrete-Time Integrator1/1
  Chart/2(Reset) -> Discrete-Time Integrator1/2
  Math Function/1 -> Chart/2(Period)
  Freq/1 -> Math Function/1
  Memory/1 -> Chart/4(IntVal)
  ResetState/1 -> Chart/1(ResetState)

== system TestStructure/Control/Tasks/LLWManualTask/Subsystem ==
  u1 : Inport
  PositiveLimit : Inport  Port=2
  Profile : Inport  Port=3
  Action Port : ActionPort  ActionPortLabel=if((u1 >= 0))
  Constant15 : Constant  Value=0
  If Action Subsystem4 : Subsystem  TreatAsAtomicUnit=on
  If Action Subsystem5 : Subsystem  TreatAsAtomicUnit=on
  If2 : If  NumInputs=2  IfExpression=(u1 <= u2)
  Merge1 : Merge
  MinMax : MinMax  Inputs=2
  Out1 : Outport
  wires:
  MinMax/1 -> If Action Subsystem4/1(In1)
  Profile/1 -> MinMax/2, If Action Subsystem5/1(In1)
  If2/1 -> If Action Subsystem5/Action
  u1/1 -> If2/1
  If2/2 -> If Action Subsystem4/Action
  If Action Subsystem5/1(Out1) -> Merge1/2
  If Action Subsystem4/1(Out1) -> Merge1/1
  PositiveLimit/1 -> If2/2
  Merge1/1 -> Out1/1
  Constant15/1 -> MinMax/1

== system TestStructure/Control/Tasks/LLWManualTask/Subsystem1 ==
  u1 : Inport
  NegtiveLimit : Inport  Port=2
  Profile : Inport  Port=3
  Action Port : ActionPort  ActionPortLabel=else
  Constant16 : Constant  Value=0
  If Action Subsystem1 : Subsystem  TreatAsAtomicUnit=on
  If Action Subsystem2 : Subsystem  TreatAsAtomicUnit=on
  If1 : If  NumInputs=2  IfExpression=(u1 >= u2)
  Merge1 : Merge
  MinMax : MinMax  Function=max  Inputs=2
  Out1 : Outport
  wires:
  Profile/1 -> MinMax/2, If Action Subsystem2/1(Motor1Pos)
  u1/1 -> If1/1
  If Action Subsystem2/1(Out1) -> Merge1/2
  If Action Subsystem1/1(Out1) -> Merge1/1
  NegtiveLimit/1 -> If1/2
  Merge1/1 -> Out1/1
  If1/2 -> If Action Subsystem1/Action
  If1/1 -> If Action Subsystem2/Action
  MinMax/1 -> If Action Subsystem1/1(In1)
  Constant16/1 -> MinMax/1

== system TestStructure/Control/Tasks/LLWManualTask/Subsystem2 ==
  u1 : Inport
  PositiveLimit : Inport  Port=2
  Profile : Inport  Port=3
  Action Port : ActionPort  ActionPortLabel=if((u1 >= 0))
  Constant15 : Constant  Value=0
  If Action Subsystem4 : Subsystem  TreatAsAtomicUnit=on
  If Action Subsystem5 : Subsystem  TreatAsAtomicUnit=on
  If2 : If  NumInputs=2  IfExpression=(u1 <= u2)
  Merge1 : Merge
  MinMax : MinMax  Inputs=2
  Out1 : Outport
  wires:
  MinMax/1 -> If Action Subsystem4/1(In1)
  Profile/1 -> MinMax/2, If Action Subsystem5/1(In1)
  If2/1 -> If Action Subsystem5/Action
  u1/1 -> If2/1
  If2/2 -> If Action Subsystem4/Action
  If Action Subsystem5/1(Out1) -> Merge1/2
  If Action Subsystem4/1(Out1) -> Merge1/1
  PositiveLimit/1 -> If2/2
  Merge1/1 -> Out1/1
  Constant15/1 -> MinMax/1

== system TestStructure/Control/Tasks/LLWManualTask/Subsystem3 ==
  u1 : Inport
  NegtiveLimit : Inport  Port=2
  Profile : Inport  Port=3
  Action Port : ActionPort  ActionPortLabel=else
  Constant16 : Constant  Value=0
  If Action Subsystem1 : Subsystem  TreatAsAtomicUnit=on
  If Action Subsystem2 : Subsystem  TreatAsAtomicUnit=on
  If1 : If  NumInputs=2  IfExpression=(u1 >= u2)
  Merge1 : Merge
  MinMax : MinMax  Function=max  Inputs=2
  Out1 : Outport
  wires:
  Profile/1 -> MinMax/2, If Action Subsystem2/1(Motor1Pos)
  u1/1 -> If1/1
  If Action Subsystem2/1(Out1) -> Merge1/2
  If Action Subsystem1/1(Out1) -> Merge1/1
  NegtiveLimit/1 -> If1/2
  Merge1/1 -> Out1/1
  If1/2 -> If Action Subsystem1/Action
  If1/1 -> If Action Subsystem2/Action
  MinMax/1 -> If Action Subsystem1/1(In1)
  Constant16/1 -> MinMax/1

== system TestStructure/Control/Tasks/PauseTask/If Action Subsystem12 ==
  In1 : Inport
  Action Port : ActionPort  ActionPortLabel=if((u1 > 4))
  Out1 : Outport
  wires:
  In1/1 -> Out1/1

== system TestStructure/Control/Tasks/PauseTask/If Action Subsystem13 ==
  In1 : Inport
  Action Port : ActionPort  ActionPortLabel=else
  Out1 : Outport
  wires:
  In1/1 -> Out1/1

== system TestStructure/Control/Tasks/StopTask/If Action Subsystem10 ==
  y : Inport
  Action Port : ActionPort  ActionPortLabel=if(u1 < -0)
  Out1 : Outport
  wires:
  y/1 -> Out1/1

== system TestStructure/Control/Tasks/StopTask/If Action Subsystem11 ==
  y : Inport
  Action Port : ActionPort  ActionPortLabel=else
  Out1 : Outport
  wires:
  y/1 -> Out1/1

== system TestStructure/Control/Tasks/StopTask/If Action Subsystem12 ==
  In1 : Inport
  Action Port : ActionPort  ActionPortLabel=if((u1 > 4))
  Out1 : Outport
  wires:
  In1/1 -> Out1/1

== system TestStructure/Control/Tasks/StopTask/If Action Subsystem13 ==
  In1 : Inport
  Action Port : ActionPort  ActionPortLabel=else
  Out1 : Outport
  wires:
  In1/1 -> Out1/1

== system TestStructure/Control/Tasks/StopTask/If Action Subsystem4 ==
  In1 : Inport
  Action Port : ActionPort  ActionPortLabel=if((u1 <= 1))
  Out1 : Outport
  wires:
  In1/1 -> Out1/1

== system TestStructure/Control/Tasks/StopTask/If Action Subsystem5 ==
  In1 : Inport
  Action Port : ActionPort  ActionPortLabel=else
  Out1 : Outport
  wires:
  In1/1 -> Out1/1

== system TestStructure/Control/Tasks/StopTask/If Action Subsystem6 ==
  In1 : Inport
  Action Port : ActionPort  ActionPortLabel=if((u1 <= 1))
  Out1 : Outport
  wires:
  In1/1 -> Out1/1

== system TestStructure/Control/Tasks/StopTask/If Action Subsystem7 ==
  In1 : Inport
  Action Port : ActionPort  ActionPortLabel=else
  Out1 : Outport
  wires:
  In1/1 -> Out1/1

== system TestStructure/Control/Tasks/StopTask/If Action Subsystem8 ==
  y : Inport
  Action Port : ActionPort  ActionPortLabel=if(u1 < -0)
  Out1 : Outport
  wires:
  y/1 -> Out1/1

== system TestStructure/Control/Tasks/StopTask/If Action Subsystem9 ==
  In1 : Inport
  Action Port : ActionPort  ActionPortLabel=else
  Out1 : Outport
  wires:
  In1/1 -> Out1/1

== system TestStructure/Control/Tasks/ULLockTask/If Action Subsystem12 ==
  In1 : Inport
  Action Port : ActionPort  ActionPortLabel=if((u1 > 4))
  Out1 : Outport
  wires:
  In1/1 -> Out1/1

== system TestStructure/Control/Tasks/ULLockTask/If Action Subsystem13 ==
  In1 : Inport
  Action Port : ActionPort  ActionPortLabel=else
  Out1 : Outport
  wires:
  In1/1 -> Out1/1

== system TestStructure/Control/Tasks/ULUnLockTask/If Action Subsystem12 ==
  In1 : Inport
  Action Port : ActionPort  ActionPortLabel=if((u1 > 4))
  Out1 : Outport
  wires:
  In1/1 -> Out1/1

== system TestStructure/Control/Tasks/ULUnLockTask/If Action Subsystem13 ==
  In1 : Inport
  Action Port : ActionPort  ActionPortLabel=else
  Out1 : Outport
  wires:
  In1/1 -> Out1/1

== system TestStructure/Control/PanelController/Display_State_1_Enable/Subsystem/Switch Case Action Subsystem ==
  In1 : Inport
  Action Port : ActionPort  ActionPortLabel=case [ 1 ]:
  Out1 : Outport
  wires:
  In1/1 -> Out1/1

== system TestStructure/Control/PanelController/Display_State_1_Enable/Subsystem/Switch Case Action Subsystem1 ==
  In1 : Inport
  Action Port : ActionPort  ActionPortLabel=default:
  Default : Outport
  wires:
  In1/1 -> Default/1

== system TestStructure/Control/PanelController/Display_State_2_Enable/Subsystem/Switch Case Action Subsystem ==
  In1 : Inport
  Action Port : ActionPort  ActionPortLabel=case [ 2 ]:
  Out1 : Outport
  wires:
  In1/1 -> Out1/1

== system TestStructure/Control/PanelController/Display_State_2_Enable/Subsystem/Switch Case Action Subsystem1 ==
  In1 : Inport
  Action Port : ActionPort  ActionPortLabel=default:
  Default : Outport
  wires:
  In1/1 -> Default/1

== system TestStructure/Control/PanelController/Display_State_3_Enable/Subsystem/Switch Case Action Subsystem ==
  In1 : Inport
  Action Port : ActionPort  ActionPortLabel=case [ 3 ]:
  Out1 : Outport
  wires:
  In1/1 -> Out1/1

== system TestStructure/Control/PanelController/Display_State_3_Enable/Subsystem/Switch Case Action Subsystem1 ==
  In1 : Inport
  Action Port : ActionPort  ActionPortLabel=default:
  Default : Outport
  wires:
  In1/1 -> Default/1

== system TestStructure/Control/PanelController/Display_State_4_Enable/Subsystem/Switch Case Action Subsystem ==
  In1 : Inport
  Action Port : ActionPort  ActionPortLabel=case [ 4 ]:
  Out1 : Outport
  wires:
  In1/1 -> Out1/1

== system TestStructure/Control/PanelController/Display_State_4_Enable/Subsystem/Switch Case Action Subsystem1 ==
  In1 : Inport
  Action Port : ActionPort  ActionPortLabel=default:
  Default : Outport
  wires:
  In1/1 -> Default/1

== system TestStructure/Control/PanelController/LLTaskControl_State_1_Enable/Subsystem/Switch Case Action Subsystem ==
  In1 : Inport
  Action Port : ActionPort  ActionPortLabel=case [ 1 ]:
  Out1 : Outport
  wires:
  In1/1 -> Out1/1

== system TestStructure/Control/PanelController/LLTaskControl_State_1_Enable/Subsystem/Switch Case Action Subsystem1 ==
  In1 : Inport
  Action Port : ActionPort  ActionPortLabel=default:
  Default : Outport
  wires:
  In1/1 -> Default/1

== system TestStructure/Control/PanelController/LLTaskControl_State_2_Enable/Subsystem/Switch Case Action Subsystem ==
  In1 : Inport
  Action Port : ActionPort  ActionPortLabel=case [ 2 ]:
  Out1 : Outport
  wires:
  In1/1 -> Out1/1

== system TestStructure/Control/PanelController/LLTaskControl_State_2_Enable/Subsystem/Switch Case Action Subsystem1 ==
  In1 : Inport
  Action Port : ActionPort  ActionPortLabel=default:
  Default : Outport
  wires:
  In1/1 -> Default/1

== system TestStructure/Control/PanelController/LLTaskControl_State_3_Enable/Subsystem/Switch Case Action Subsystem ==
  In1 : Inport
  Action Port : ActionPort  ActionPortLabel=case [ 3 ]:
  Out1 : Outport
  wires:
  In1/1 -> Out1/1

== system TestStructure/Control/PanelController/LLTaskControl_State_3_Enable/Subsystem/Switch Case Action Subsystem1 ==
  In1 : Inport
  Action Port : ActionPort  ActionPortLabel=default:
  Default : Outport
  wires:
  In1/1 -> Default/1

== system TestStructure/Control/PanelController/LLTaskControl_State_4_Enable/Subsystem/Switch Case Action Subsystem ==
  In1 : Inport
  Action Port : ActionPort  ActionPortLabel=case [ 4 ]:
  Out1 : Outport
  wires:
  In1/1 -> Out1/1

== system TestStructure/Control/PanelController/LLTaskControl_State_4_Enable/Subsystem/Switch Case Action Subsystem1 ==
  In1 : Inport
  Action Port : ActionPort  ActionPortLabel=default:
  Default : Outport
  wires:
  In1/1 -> Default/1

== system TestStructure/Control/PanelController/LLTaskControl_State_5_Enable/Subsystem/Switch Case Action Subsystem ==
  In1 : Inport
  Action Port : ActionPort  ActionPortLabel=case [ 5 ]:
  Out1 : Outport
  wires:
  In1/1 -> Out1/1

== system TestStructure/Control/PanelController/LLTaskControl_State_5_Enable/Subsystem/Switch Case Action Subsystem1 ==
  In1 : Inport
  Action Port : ActionPort  ActionPortLabel=default:
  Default : Outport
  wires:
  In1/1 -> Default/1

== system TestStructure/Control/PanelController/LLTaskControl_State_6_Enable/Subsystem/Switch Case Action Subsystem ==
  In1 : Inport
  Action Port : ActionPort  ActionPortLabel=case [ 6 ]:
  Out1 : Outport
  wires:
  In1/1 -> Out1/1

== system TestStructure/Control/PanelController/LLTaskControl_State_6_Enable/Subsystem/Switch Case Action Subsystem1 ==
  In1 : Inport
  Action Port : ActionPort  ActionPortLabel=default:
  Default : Outport
  wires:
  In1/1 -> Default/1

== system TestStructure/Control/PanelController/LLTaskControl_State_7_Enable/Subsystem/Switch Case Action Subsystem ==
  In1 : Inport
  Action Port : ActionPort  ActionPortLabel=case [ 7 ]:
  Out1 : Outport
  wires:
  In1/1 -> Out1/1

== system TestStructure/Control/PanelController/LLTaskControl_State_7_Enable/Subsystem/Switch Case Action Subsystem1 ==
  In1 : Inport
  Action Port : ActionPort  ActionPortLabel=default:
  Default : Outport
  wires:
  In1/1 -> Default/1

== system TestStructure/Control/PanelController/LLTaskControl_State_8_Enable/Subsystem/Switch Case Action Subsystem ==
  In1 : Inport
  Action Port : ActionPort  ActionPortLabel=case [ 8 ]:
  Out1 : Outport
  wires:
  In1/1 -> Out1/1

== system TestStructure/Control/PanelController/LLTaskControl_State_8_Enable/Subsystem/Switch Case Action Subsystem1 ==
  In1 : Inport
  Action Port : ActionPort  ActionPortLabel=default:
  Default : Outport
  wires:
  In1/1 -> Default/1

== system TestStructure/Control/PanelController/LLTaskControl_State_9_Enable/Subsystem/Switch Case Action Subsystem ==
  In1 : Inport
  Action Port : ActionPort  ActionPortLabel=case [ 9 ]:
  Out1 : Outport
  wires:
  In1/1 -> Out1/1

== system TestStructure/Control/PanelController/LLTaskControl_State_9_Enable/Subsystem/Switch Case Action Subsystem1 ==
  In1 : Inport
  Action Port : ActionPort  ActionPortLabel=default:
  Default : Outport
  wires:
  In1/1 -> Default/1

== system TestStructure/Control/PanelController/ULTaskControl_State_1_Enable/Subsystem/Switch Case Action Subsystem ==
  In1 : Inport
  Action Port : ActionPort  ActionPortLabel=case [ 1 ]:
  Out1 : Outport
  wires:
  In1/1 -> Out1/1

== system TestStructure/Control/PanelController/ULTaskControl_State_1_Enable/Subsystem/Switch Case Action Subsystem1 ==
  In1 : Inport
  Action Port : ActionPort  ActionPortLabel=default:
  Default : Outport
  wires:
  In1/1 -> Default/1

== system TestStructure/Control/PanelController/ULTaskControl_State_2_Enable/Subsystem/Switch Case Action Subsystem ==
  In1 : Inport
  Action Port : ActionPort  ActionPortLabel=case [ 2 ]:
  Out1 : Outport
  wires:
  In1/1 -> Out1/1

== system TestStructure/Control/PanelController/ULTaskControl_State_2_Enable/Subsystem/Switch Case Action Subsystem1 ==
  In1 : Inport
  Action Port : ActionPort  ActionPortLabel=default:
  Default : Outport
  wires:
  In1/1 -> Default/1

== system TestStructure/Control/Tasks/LLBManualTask/Subsystem/If Action Subsystem4 ==
  In1 : Inport
  Action Port : ActionPort  ActionPortLabel=else
  Out1 : Outport
  wires:
  In1/1 -> Out1/1

== system TestStructure/Control/Tasks/LLBManualTask/Subsystem/If Action Subsystem5 ==
  In1 : Inport
  Action Port : ActionPort  ActionPortLabel=if((u1 <= u2))
  Out1 : Outport
  wires:
  In1/1 -> Out1/1

== system TestStructure/Control/Tasks/LLBManualTask/Subsystem1/If Action Subsystem1 ==
  In1 : Inport
  Action Port : ActionPort  ActionPortLabel=else
  Out1 : Outport
  wires:
  In1/1 -> Out1/1
